simulink model "Force"  (R2017b)
settings: Solver=VariableStepAuto  StartTime=0.0  StopTime=10.0  RelTol=1e-3
settings Model: Creator=Kalana  LastModifiedBy=Kalana

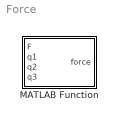
== system Force ==
  MATLAB Function : MATLAB Function  TreatAsAtomicUnit=on

== matlab function Force/MATLAB Function ==
  data: F input; force output; q1 input; q2 input; q3 input
function force = Force(F, q1, q2, q3)

JvEE = [-0.245*sin(q1)*cos(q2-q3)-0.2*sin(q1)*cos(q2)-0.1225*sin(q1)+0.0525*cos(q1),  -0.245*cos(q1)*sin(q2-q3)-0.2*cos(q1)*sin(q2),  0.245*cos(q1)*sin(q2-q3);
        0.245*cos(q1)*cos(q2-q3)+0.2*cos(q1)*cos(q2)+0.1225*cos(q1)+0.0525*sin(q1),   -0.245*sin(q1)*sin(q2-q3)-0.2*sin(q1)*sin(q2),  0.245*sin(q1)*sin(q2-q3);
        0,                                                                            -0.245*cos(q2-q3)-0.2*cos(q2),                  0.245*cos(q2-q3)       ];

force = JvEE'*F;
